simulink model "counter_up"  (R2021a)
settings: Solver=FixedStepDiscrete  StartTime=0.0  StopTime=100  RelTol=1e-3  EnableMultiTasking=on
settings Model: Creator=iT-User  LastModifiedBy=iT-User
settings DataIOCC: ReturnWorkspaceOutputs=off
settings OptimizationCC: DefaultParameterBehavior=Inlined  InlineInvariantSignals=on  EnableMemcpy=off  LifeSpan=1  EfficientTunableParamExpr=on
settings DebuggingCC: UnderspecifiedInitializationDetection=Classic  MergeDetectMultiDrivingBlocksExec=none  SFMachineParentedDataDiag=warning  ArithmeticOperatorsInVariantConditions=warning
settings ModelReferenceCC: PropagateSignalLabelsOutOfModel=off
settings SFSimCC: MATLABDynamicMemAlloc=off  CustomCodeUndefinedFunction=UseInterfaceOnly
settings RTWCC: SystemTargetFile=ert.tlc  GenCodeOnly=on  TemplateMakefile=ert_default_tmf  GenerateReport=on  IncludeHyperlinkInReport=on  LaunchReport=on  GenerateTraceInfo=on  GenerateTraceReport=on  GenerateTraceReportSl=on  GenerateTraceReportSf=on  GenerateTraceReportEml=on
settings CodeAppCC: ForceParamTrailComments=on  IgnoreCustomStorageClasses=off  OperatorAnnotations=on  SimulinkDataObjDesc=on  SFDataObjDesc=on  MATLABFcnDesc=on  InsertBlockDesc=on  StateflowObjectComments=on  MATLABSourceComments=on
settings ERTTargetCC: MultiwordLength=2048  GenerateSampleERTMain=on  InlinedParameterPlacement=NonHierarchical  ERTCustomFileTemplate=example_file_process.tlc

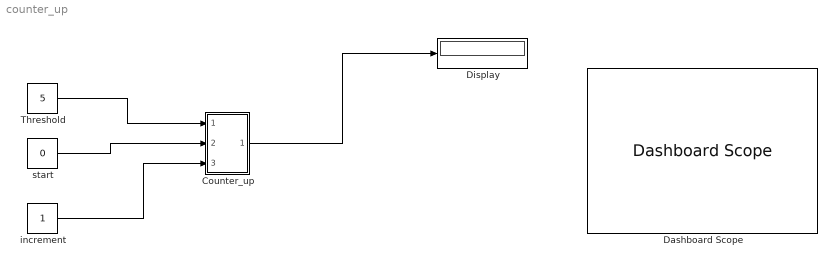
== system counter_up ==
  Counter_up : Subsystem
  Dashboard Scope : DashboardScope  Ymin=0  Ymax=6  NormalizeYAxis=on
  Display : Display
  Threshold : Constant  Value=5
  increment : Constant
  start : Constant  Value=0
  wires:
  Threshold/1 -> Counter_up/1(In1)
  start/1 -> Counter_up/2(In2)
  increment/1 -> Counter_up/3(In3)
  Counter_up/1(Out1) -> Display/1

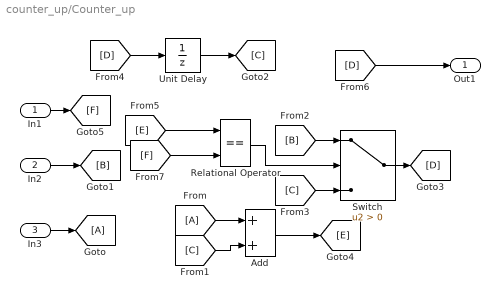
== system counter_up/Counter_up ==
  In1 : Inport
  In2 : Inport  Port=2
  In3 : Inport  Port=3
  Add : Sum
  Relational Operator : RelationalOperator  Operator===  OutDataTypeStr=boolean  RndMeth=Simplest
  Switch : Switch  Criteria=u2 > Threshold
  Unit Delay : UnitDelay  HasFrameUpgradeWarning=on
  Out1 : Outport
  wires:
  [C] -> Add/2
  Unit Delay/1 -> [C]
  [B] -> Switch/1
  Add/1 -> [E]
  [A] -> Add/1
  [F] -> Relational Operator/2
  [C] -> Switch/3
  Relational Operator/1 -> Switch/2
  [E] -> Relational Operator/1
  [D] -> Unit Delay/1
  Switch/1 -> [D]
  In3/1 -> [A]
  [D] -> Out1/1
  In1/1 -> [F]
  In2/1 -> [B]
